simulink model "Newton_Euler_1_D"  (R2023b)
settings: Solver=FixedStepAuto  StartTime=0.0  StopTime=15  RelTol=1e-3  AbsTol=1e-3  EnableMultiTasking=on
model workspace (MAT data in the model file):
  l1 = 20
  m1 = 1
undefined symbols (not defined in the file): X, Y, Z
libraries: sm_lib x13, nesl_utility x13, robotcorelib x1, simulink x1
settings Model: Creator=digimax  LastModifiedBy=digimax
settings SolverCC: AutoScaleAbsTol=off  AlgebraicLoopSolver=TrustRegion  MaxZcPerStep=1
settings DataIOCC: LimitDataPoints=on  MaxDataPoints=10000
settings OptimizationCC: ReuseModelBlockBuffer=off  LifeSpan=inf
settings DebuggingCC: UnconnectedInputMsg=warning  UnconnectedOutputMsg=warning  UnconnectedLineMsg=warning  AllowSymbolicDim=off  SFUnexpectedBacktrackingDiag=warning  SFNoUnconditionalDefaultTransitionDiag=warning  SFExecutionAtInitializationDiag=none  ArithmeticOperatorsInVariantConditions=warning
settings ModelReferenceCC: EnableRefExpFcnMdlSchedulingChecks=on
settings SFSimCC: SimUseLocalCustomCode=off  CustomCodeUndefinedFunction=UseInterfaceOnly
settings RTWCC: RTWUseLocalCustomCode=off  DLArmComputeVersion=19.05
settings CodeAppCC: StateflowObjectComments=on
settings GRTTargetCC: TargetLangStandard=C89/C90 (ANSI)
settings ConfigComp: CovMetricSettings=dw  CovSaveCumulativeToWorkspaceVar=on  CovSaveSingleToWorkspaceVar=on  CovExternalEMLEnable=off  CovSFcnEnable=off
settings SimscapeCC: SimscapeLogType=all  SimscapeLogSimulationStatistics=on  SimscapeLogDataHistory=10000

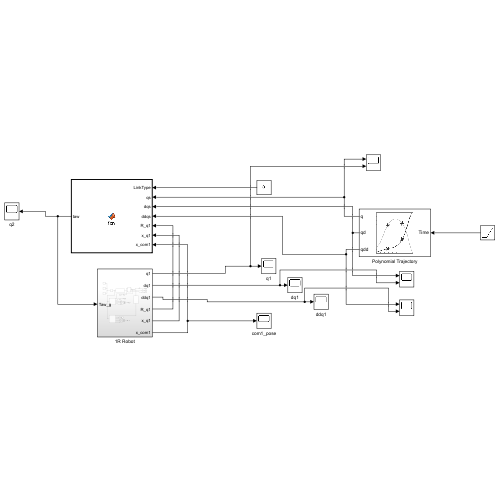
[thumbnail: Simulink's stored preview of the top-level diagram]
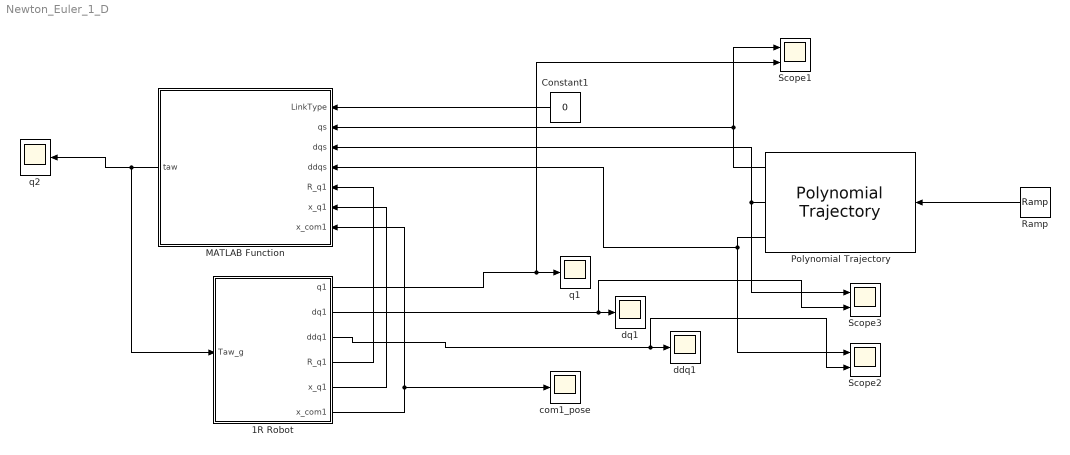
== system Newton_Euler_1_D ==
  1R Robot : Subsystem
  Constant1 : Constant  Value=0
  MATLAB Function : MATLAB Function  TreatAsAtomicUnit=on
  Polynomial Trajectory : robotcorelib/Polynomial Trajectory  WaypointSource=Internal  Waypoints=[ 0, pi/6,-pi/6 ]  TimePoints=[ 0, 5,10]  TimeInterval=[ 1, 4 ]  Method=Cubic Polynomial  ParameterSource=Internal  VelocityBoundaryCondition=zeros( 1, 3)  AccelerationBoundaryCondition=zeros( 2, 5 )  SimulateUsing=Interpreted execution
  Ramp : simulink/Sources/Ramp  slope=1  start=0  InitialOutput=0
  Scope1 : Scope  NumInputPorts=2
  Scope2 : Scope  NumInputPorts=2
  Scope3 : Scope  NumInputPorts=2
  com1_pose : Scope
  ddq1 : Scope
  dq1 : Scope
  q1 : Scope
  q2 : Scope
  wires:
  1R Robot/1(q1) -> Scope1/2, q1/1
  1R Robot/6(x_com1) -> MATLAB Function/7(x_com1), com1_pose/1
  1R Robot/4(R_q1) -> MATLAB Function/5(R_q1)
  1R Robot/5(x_q1) -> MATLAB Function/6(x_q1)
  1R Robot/2(dq1) -> Scope3/2, dq1/1
  Constant1/1 -> MATLAB Function/1(LinkType)
  Ramp/1 -> Polynomial Trajectory/1
  Polynomial Trajectory/1 -> MATLAB Function/2(qs), Scope1/1
  Polynomial Trajectory/2 -> MATLAB Function/3(dqs), Scope3/1
  1R Robot/3(ddq1) -> Scope2/2, ddq1/1
  Polynomial Trajectory/3 -> MATLAB Function/4(ddqs), Scope2/1
  MATLAB Function/1(taw) -> 1R Robot/1(Taw_g), q2/1

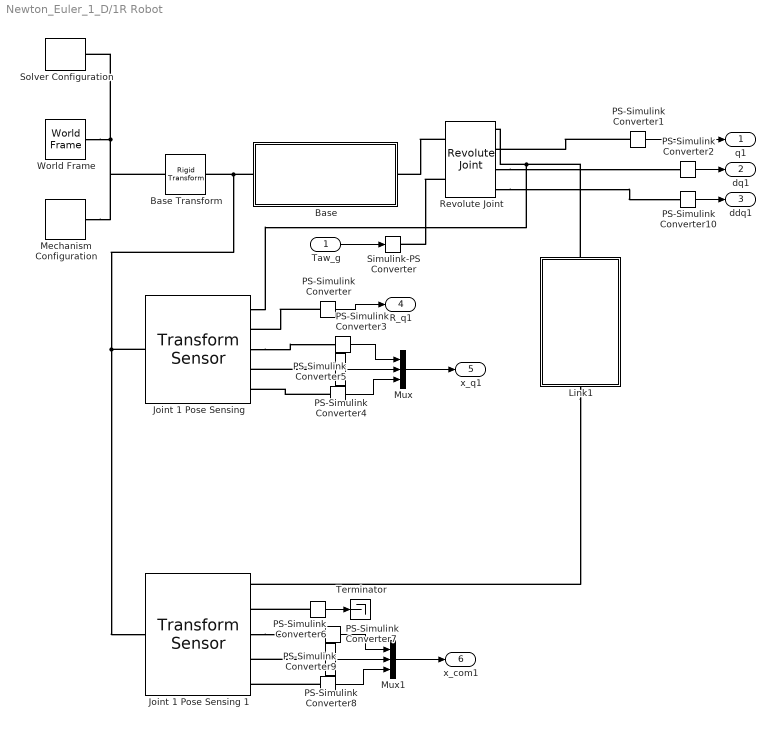
== system Newton_Euler_1_D/1R Robot ==
  Taw_g : Inport
  Base : Subsystem
  Base Transform : sm_lib/Frames and Transforms/Rigid Transform  TranslationMethod=None  TranslationStandardOffset=0  TranslationStandardOffsetUnits=m  TranslationStandardAxis=+Z  TranslationCartesianOffset=[0 0 0]  TranslationCartesianOffsetUnits=m  TranslationROffset=0  TranslationROffsetUnits=m  TranslationZOffset=0  TranslationZOffsetUnits=m  TranslationThetaOffset=0  TranslationThetaOffsetUnits=deg  RotationMethod=AlignedAxes  RotationAngleUnits=deg  RotationStandardAxis=+Z  RotationAngle=0.0  RotationArbitraryAxis=[0 0 1]  FollAlignAxisA=+Z  BaseAlignAxisA=-Y  FollAlignAxisB=+X  BaseAlignAxisB=+X  RotationSequenceAxes=FollowerAxes  RotationSequence=XYX  RotationSequenceAngles=[0 0 0]  RotationSequenceAnglesUnits=deg  RotationMatrix=[1 0 0; 0 1 0; 0 0 1]  Quaternion=[1 0 0 0]
  "Joint 1 Pose Sensing " : sm_lib/Frames and Transforms/Transform Sensor  MeasurementFrame=Base  RotationSequence=XYX  SenseAngle=off  SenseAxis=off  SenseQ=off  SenseR=on  SenseRotationSequence=off  SenseOmegaX=off  SenseOmegaY=off  SenseOmegaZ=off  SenseOmega=off  SenseQDot=off  SenseRDot=off  SenseRotationSequenceDot=off  SenseAlphaX=off  SenseAlphaY=off  SenseAlphaZ=off  SenseAlpha=off  SenseQDDot=off  SenseRDDot=off  SenseX=on  SenseY=on  SenseZ=on  SenseXYZ=off  SenseRad=off  SenseAzim=off  SenseDist=off  SenseInc=off  SenseXDot=off  SenseYDot=off  SenseZDot=off  SenseXYZDot=off  SenseRadDot=off  SenseAzimDot=off  SenseDistDot=off  SenseIncDot=off  SenseXDDot=off  SenseYDDot=off  SenseZDDot=off  SenseXYZDDot=off  SenseRadDDot=off  SenseAzimDDot=off  SenseDistDDot=off  SenseIncDDot=off
  Joint 1 Pose Sensing 1 : sm_lib/Frames and Transforms/Transform Sensor  MeasurementFrame=Base  RotationSequence=XYX  SenseAngle=off  SenseAxis=off  SenseQ=off  SenseR=on  SenseRotationSequence=off  SenseOmegaX=off  SenseOmegaY=off  SenseOmegaZ=off  SenseOmega=off  SenseQDot=off  SenseRDot=off  SenseRotationSequenceDot=off  SenseAlphaX=off  SenseAlphaY=off  SenseAlphaZ=off  SenseAlpha=off  SenseQDDot=off  SenseRDDot=off  SenseX=on  SenseY=on  SenseZ=on  SenseXYZ=off  SenseRad=off  SenseAzim=off  SenseDist=off  SenseInc=off  SenseXDot=off  SenseYDot=off  SenseZDot=off  SenseXYZDot=off  SenseRadDot=off  SenseAzimDot=off  SenseDistDot=off  SenseIncDot=off  SenseXDDot=off  SenseYDDot=off  SenseZDDot=off  SenseXYZDDot=off  SenseRadDDot=off  SenseAzimDDot=off  SenseDistDDot=off  SenseIncDDot=off
  Link1 : Subsystem
  Mechanism Configuration : sm_lib/Utilities/Mechanism Configuration  UniformGravity=Constant  GravityVector=[0 0 -9.81]  GravityVectorUnits=m/s^2  LinearizationDelta=0.001  JointModeTransitionNonlinearIterations=2
  Mux : Mux  Inputs=3
  Mux1 : Mux  Inputs=3
  PS-Simulink Converter{,1..10} (11 alike) : nesl_utility/PS-Simulink Converter  PhysicalDomain=network_engine_domain  SubClassName=ps_output  LeftPortType=input  RightPortType=output  PseudoPeriodic=off  Frequencies=[]  VectorFormat=inherit  Unit=inherit  AffineConversion=off
  Revolute Joint : sm_lib/Joints/Revolute Joint  JointMode=Normal  SenseConstraintForce=off  SenseConstraintForceX=off  SenseConstraintForceY=off  SenseConstraintForceZ=off  SenseConstraintTorque=off  SenseConstraintTorqueX=off  SenseConstraintTorqueY=off  SenseConstraintTorqueZ=off  SenseTotalForce=off  SenseTotalForceX=off  SenseTotalForceY=off  SenseTotalForceZ=off  SenseTotalTorque=off  SenseTotalTorqueX=off  SenseTotalTorqueY=off  SenseTotalTorqueZ=off  CompositeWrenchDir=FollowerOnBase  CompositeWrenchFrame=BaseFrame  EquilibriumPosition=0  EquilibriumPositionUnits=deg  SpringStiffness=0  SpringStiffnessUnits=N*m/deg  DampingCoefficient=0  DampingCoefficientUnits=N*m/(deg/s)  TorqueActuationMode=InputTorque  MotionActuationMode=ComputedMotion  SensePosition=on  SenseVelocity=on  SenseAcceleration=on  SenseTorqueForce=off  SenseLowerLimitTorqueForce=off  SenseUpperLimitTorqueForce=off  LowerLimitSpecify=off  LowerLimitBound=-90  LowerLimitBoundUnits=deg  LowerLimitStiffness=1e4  LowerLimitStiffnessUnits=N*m/deg  LowerLimitDamping=10  LowerLimitDampingUnits=N*m/(deg/s)  LowerLimitTransitionRegionWidth=0.1  LowerLimitTransitionRegionWidthUnits=deg  UpperLimitSpecify=off  UpperLimitBound=90  UpperLimitBoundUnits=deg  UpperLimitStiffness=1e4  UpperLimitStiffnessUnits=N*m/deg  UpperLimitDamping=10  UpperLimitDampingUnits=N*m/(deg/s)  UpperLimitTransitionRegionWidth=0.1  UpperLimitTransitionRegionWidthUnits=deg  PositionTargetSpecify=on  PositionTargetPriority=High  PositionTargetValue=0  PositionTargetValueUnits=deg  VelocityTargetSpecify=off  VelocityTargetPriority=High  VelocityTargetValue=0  VelocityTargetValueUnits=deg/s
  Simulink-PS Converter : nesl_utility/Simulink-PS Converter  PhysicalDomain=network_engine_domain  SubClassName=ps_input  LeftPortType=input  RightPortType=output  PseudoPeriodic=off  Frequencies=[]  NoiseDistribution=none  NoiseParameters=[]  Unit=1  AffineConversion=off  FilteringAndDerivatives=provide  SimscapeFilterOrder=1  InputFilterTimeConstant=0.001  UdotUserProvided=0
  Solver Configuration : nesl_utility/Solver Configuration  PhysicalDomain=network_engine_domain  SubClassName=solver  LeftPortType=input  RightPortType=generic  Tones=[]  Harmonics=[]  SimulateNoise=off  Profile=off  UseLocalSampling=off  EnableSwitchedLinearOptims=on  FrequencyDomain=off  UseCCode=off  RelTol=0.001  AbsTol=1e-06  MinStep=1e-09  ToWorkspace=off  RevertToSquareIcSolve=off  NumHomotopyIterations=100  PhasorMode=off  PhasorModeNumHarmonics=1  ConsistencySolver=NEWTON_XTOL_AFTER_FTOL  IndexReductionMethod=DerivativeReplacement  DoDC=off  ResidualTolerance=1e-09  ConsistencyTolSource=GLOBAL  ConsistencyAbsTol=0.001  ConsistencyRelTol=0.001  ConsistencyTolFactor=0.001  UseLocalSolver=off  LocalSolverChoice=NE_BACKWARD_EULER_ADVANCER  ResolveIndetEquations=on  FunctionEvalNumThread=1  LocalSolverSampleTime=0.001  DoFixedCost=off  MaxNonlinIter=3  MaxModeIter=2  ComputeImpulses=off  ImpulseIterations=2  LinearAlgebra=Sparse  LinearAlgebraNumThread=0  EquationFormulation=NE_TIME_EF  DelaysMemoryBudget=1024  AutomaticFiltering=on  FilteringTimeConstant=0.001  PartitionStorageMethod=AS_NEEDED  PartitionMemoryBudget=1024  PartitionMethod=FAST  MultibodyUseLocalSolver=off  MultibodyLocalSolverChoice=ODE1  MultibodyLocalSolverSampleTime=0.001
  Terminator : Terminator
  World Frame : sm_lib/Frames and Transforms/World Frame
  q1 : Outport
  dq1 : Outport  Port=2
  ddq1 : Outport  Port=3
  R_q1 : Outport  Port=4
  x_q1 : Outport  Port=5
  x_com1 : Outport  Port=6
  wires:
  PS-Simulink Converter1/1 -> q1/1
  Taw_g/1 -> Simulink-PS Converter/1
  PS-Simulink Converter/1 -> R_q1/1
  PS-Simulink Converter3/1 -> Mux/1
  PS-Simulink Converter4/1 -> Mux/2
  PS-Simulink Converter5/1 -> Mux/3
  Mux/1 -> x_q1/1
  Mux1/1 -> x_com1/1
  PS-Simulink Converter9/1 -> Mux1/3
  PS-Simulink Converter8/1 -> Mux1/2
  PS-Simulink Converter7/1 -> Mux1/1
  PS-Simulink Converter6/1 -> Terminator/1
  PS-Simulink Converter10/1 -> ddq1/1
  PS-Simulink Converter2/1 -> dq1/1
  connections:
  Revolute Joint/LConn1 -- Base/RConn1
  PS-Simulink Converter1/LConn1 -- Revolute Joint/RConn2
  Link1/LConn1 -- Revolute Joint/RConn1 -- "Joint 1 Pose Sensing "/RConn1
  Revolute Joint/LConn2 -- Simulink-PS Converter/RConn1
  PS-Simulink Converter/LConn1 -- "Joint 1 Pose Sensing "/RConn2
  "Joint 1 Pose Sensing "/RConn3 -- PS-Simulink Converter3/LConn1
  PS-Simulink Converter4/LConn1 -- "Joint 1 Pose Sensing "/RConn4
  PS-Simulink Converter8/LConn1 -- Joint 1 Pose Sensing 1/RConn4
  PS-Simulink Converter9/LConn1 -- Joint 1 Pose Sensing 1/RConn5
  PS-Simulink Converter6/LConn1 -- Joint 1 Pose Sensing 1/RConn2
  Joint 1 Pose Sensing 1/RConn3 -- PS-Simulink Converter7/LConn1
  Link1/RConn1 -- Joint 1 Pose Sensing 1/RConn1
  PS-Simulink Converter5/LConn1 -- "Joint 1 Pose Sensing "/RConn5
  World Frame/RConn1 -- Base Transform/LConn1 -- Mechanism Configuration/RConn1 -- Solver Configuration/RConn1
  Base/LConn1 -- Joint 1 Pose Sensing 1/LConn1 -- "Joint 1 Pose Sensing "/LConn1 -- Base Transform/RConn1
  Revolute Joint/RConn3 -- PS-Simulink Converter2/LConn1
  Revolute Joint/RConn4 -- PS-Simulink Converter10/LConn1

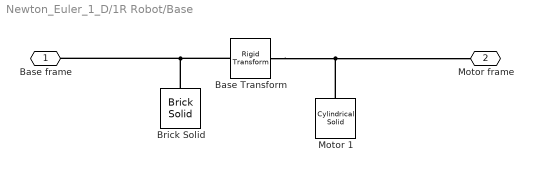
== system Newton_Euler_1_D/1R Robot/Base ==
  Base Transform : sm_lib/Frames and Transforms/Rigid Transform  TranslationMethod=StandardAxis  TranslationStandardOffset=2  TranslationStandardOffsetUnits=m  TranslationStandardAxis=+Z  TranslationCartesianOffset=[0 0 0]  TranslationCartesianOffsetUnits=m  TranslationROffset=0  TranslationROffsetUnits=m  TranslationZOffset=0  TranslationZOffsetUnits=m  TranslationThetaOffset=0  TranslationThetaOffsetUnits=deg  RotationMethod=None  RotationAngleUnits=deg  RotationStandardAxis=+Z  RotationAngle=0.0  RotationArbitraryAxis=[0 0 1]  FollAlignAxisA=+Z  BaseAlignAxisA=-Y  FollAlignAxisB=+X  BaseAlignAxisB=+X  RotationSequenceAxes=FollowerAxes  RotationSequence=XYX  RotationSequenceAngles=[0 0 0]  RotationSequenceAnglesUnits=deg  RotationMatrix=[1 0 0; 0 1 0; 0 0 1]  Quaternion=[1 0 0 0]
  Brick Solid : sm_lib/Body Elements/Brick Solid  GraphicAmbientColor=[0.15 0.15 0.15 1.0]  BasedOnType=Mass  BrickDimensions=[10 10 1]  BrickDimensionsUnits=m  CenterOfMass=[0 0 0]  CenterOfMassUnits=m  GraphicDiffuseColor=[0.5 0.5 0.5]  Density=1000  DensityUnits=kg/m^3  DoExposeReferenceFrame=on  GraphicEmissiveColor=[0.0 0.0 0.0 1.0]  ExportEntireGeometry=off  SerializedFrames=<Frames/>  MarkerShape=Sphere  MarkerSize=10  GraphicType=FromGeometry  InertiaType=CalculateFromGeometry  Mass=1  MassUnits=kg  MomentsOfInertia=[1 1 1]  MomentsOfInertiaUnits=kg*m^2  GraphicOpacity=1.0  ProductsOfInertia=[0 0 0]  ProductsOfInertiaUnits=kg*m^2  GraphicShininess=75  GraphicSpecularColor=[0.5 0.5 0.5 1.0]  GraphicVisPropType=SimpleVisualProperties
  Motor 1 : sm_lib/Body Elements/Cylindrical Solid  GraphicAmbientColor=[0.15 0.15 0.15 1.0]  BasedOnType=Mass  CenterOfMass=[0 0 0]  CenterOfMassUnits=m  GraphicDiffuseColor=[0.4 0.4 0.4]  CylinderLength=3  CylinderLengthUnits=m  CylinderRadius=1  CylinderRadiusUnits=m  Density=1000  DensityUnits=kg/m^3  DoExposeReferenceFrame=on  GraphicEmissiveColor=[0.0 0.0 0.0 1.0]  ExportEntireGeometry=off  SerializedFrames=<Frames/>  MarkerShape=Sphere  MarkerSize=10  GraphicType=FromGeometry  InertiaType=CalculateFromGeometry  Mass=1  MassUnits=kg  MomentsOfInertia=[1 1 1]  MomentsOfInertiaUnits=kg*m^2  GraphicOpacity=1.0  ProductsOfInertia=[0 0 0]  ProductsOfInertiaUnits=kg*m^2  GraphicShininess=75  GraphicSpecularColor=[0.5 0.5 0.5 1.0]  GraphicVisPropType=SimpleVisualProperties
  Base frame : PMIOPort  Side=Left
  Motor frame : PMIOPort  Port=2  Side=Right
  connections:
  Brick Solid/RConn1 -- Base Transform/LConn1 -- Base frame/RConn1
  Base Transform/RConn1 -- Motor 1/RConn1 -- Motor frame/RConn1

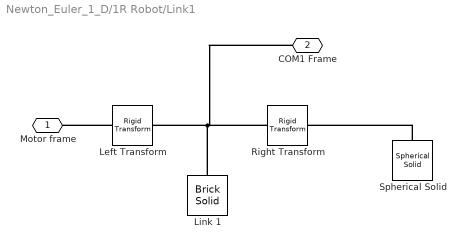
== system Newton_Euler_1_D/1R Robot/Link1 ==
  Left Transform : sm_lib/Frames and Transforms/Rigid Transform  TranslationMethod=StandardAxis  TranslationStandardOffset=10  TranslationStandardOffsetUnits=m  TranslationStandardAxis=+X  TranslationCartesianOffset=[0 0 0]  TranslationCartesianOffsetUnits=m  TranslationROffset=0  TranslationROffsetUnits=m  TranslationZOffset=0  TranslationZOffsetUnits=m  TranslationThetaOffset=0  TranslationThetaOffsetUnits=deg  RotationMethod=None  RotationAngleUnits=deg  RotationStandardAxis=+Z  RotationAngle=0.0  RotationArbitraryAxis=[0 0 1]  FollAlignAxisA=+Z  BaseAlignAxisA=-Y  FollAlignAxisB=+X  BaseAlignAxisB=+X  RotationSequenceAxes=FollowerAxes  RotationSequence=XYX  RotationSequenceAngles=[0 0 0]  RotationSequenceAnglesUnits=deg  RotationMatrix=[1 0 0; 0 1 0; 0 0 1]  Quaternion=[1 0 0 0]
  Link 1 : sm_lib/Body Elements/Brick Solid  GraphicAmbientColor=[0.15 0.15 0.15 1.0]  BasedOnType=Mass  BrickDimensions=[20 1 1]  BrickDimensionsUnits=m  CenterOfMass=[0 0 0]  CenterOfMassUnits=m  GraphicDiffuseColor=[1.0 0.0 0.0]  Density=1000  DensityUnits=kg/m^3  DoExposeReferenceFrame=on  GraphicEmissiveColor=[0.0 0.0 0.0 1.0]  ExportEntireGeometry=off  SerializedFrames=<Frames/>  MarkerShape=Sphere  MarkerSize=10  GraphicType=FromGeometry  InertiaType=CalculateFromGeometry  Mass=1  MassUnits=kg  MomentsOfInertia=[1 1 1]  MomentsOfInertiaUnits=kg*m^2  GraphicOpacity=1.0  ProductsOfInertia=[0 0 0]  ProductsOfInertiaUnits=kg*m^2  GraphicShininess=75  GraphicSpecularColor=[0.5 0.5 0.5 1.0]  GraphicVisPropType=SimpleVisualProperties
  "Right Transform " : sm_lib/Frames and Transforms/Rigid Transform  TranslationMethod=StandardAxis  TranslationStandardOffset=10  TranslationStandardOffsetUnits=m  TranslationStandardAxis=+X  TranslationCartesianOffset=[0 0 0]  TranslationCartesianOffsetUnits=m  TranslationROffset=0  TranslationROffsetUnits=m  TranslationZOffset=0  TranslationZOffsetUnits=m  TranslationThetaOffset=0  TranslationThetaOffsetUnits=deg  RotationMethod=None  RotationAngleUnits=deg  RotationStandardAxis=+Z  RotationAngle=0.0  RotationArbitraryAxis=[0 0 1]  FollAlignAxisA=+Z  BaseAlignAxisA=-Y  FollAlignAxisB=+X  BaseAlignAxisB=+X  RotationSequenceAxes=FollowerAxes  RotationSequence=XYX  RotationSequenceAngles=[0 0 0]  RotationSequenceAnglesUnits=deg  RotationMatrix=[1 0 0; 0 1 0; 0 0 1]  Quaternion=[1 0 0 0]
  Spherical Solid : sm_lib/Body Elements/Spherical Solid  GraphicAmbientColor=[0.15 0.15 0.15 1.0]  BasedOnType=Mass  CenterOfMass=[0 0 0]  CenterOfMassUnits=m  GraphicDiffuseColor=[0.0 0.0 0.8]  Density=1000  DensityUnits=kg/m^3  DoExposeReferenceFrame=on  GraphicEmissiveColor=[0.0 0.0 0.0 1.0]  ExportEntireGeometry=off  SerializedExposedGeometries=<ExposedGeometries/>  SerializedFrames=<Frames/>  MarkerShape=Sphere  MarkerSize=10  GraphicType=FromGeometry  InertiaType=CalculateFromGeometry  Mass=0  MassUnits=kg  MomentsOfInertia=[1 1 1]  MomentsOfInertiaUnits=kg*m^2  GraphicOpacity=1.0  ProductsOfInertia=[0 0 0]  ProductsOfInertiaUnits=kg*m^2  GraphicShininess=75  GraphicSpecularColor=[0.5 0.5 0.5 1.0]  SphereRadius=1  SphereRadiusUnits=m  GraphicVisPropType=SimpleVisualProperties
  Motor frame : PMIOPort  Side=Left
  COM1 Frame : PMIOPort  Port=2  Side=Right
  connections:
  Link 1/RConn1 -- "Right Transform "/LConn1 -- COM1 Frame/RConn1 -- Left Transform/RConn1
  Left Transform/LConn1 -- Motor frame/RConn1
  Spherical Solid/RConn1 -- "Right Transform "/RConn1

== matlab function Newton_Euler_1_D/MATLAB Function ==
  data: LinkType input; qs input; dqs input; ddqs input; R_q1 input; x_q1 input; x_com1 input; taw output
function taw = fcn(LinkType , qs , dqs, ddqs , R_q1 , x_q1 , x_com1)

    % Characteristics 
    linkType = [0;LinkType] ; 

    Link_num = length(LinkType) ;   % Number of Links
 
    m = zeros(Link_num+1 , 1) ;    % Vector of link masses
    m(2) = 1 ; % unit kg

    g = 9.81 ; 

    % dimensions of the links in its body frame 
    x= 20;
    y = 1 ; 
    z = 1 ; 


    Ix = m(2)/12*(x^2) ; 
    Iy = m(2)/12*(x^2) ;
    Iz = m(2)/12*(x^2) ;

    Ic1_1 = [Ix 0 0;
            0 Iy 0;
            0 0 Iz] ; 

    Ic_i = zeros(3,3,Link_num+1) ;  % matrix of inertias in the frame connected to its joint
    Ic_i(:,:,2) = Ic1_1 ; 

    
    %% Initialization 

    ri_0_0 = [zeros(3,1),x_q1];                             % Position of Joint i w.r.t base frame represented in base frame  
    r_ci_0_0 = [zeros(3,1),x_com1] ;                        % Position of Link i C.M w.r.t base frame represented in base frame  
    r_i_i_1_0 = zeros(3,Link_num+1) ;                       % Position of Joint i w.r.t Joint i-1 represented in base frame
    P_ci_i_0 = zeros(3,Link_num+1) ;

    % Matrices of Rotation
    R0_i =  zeros(3,3,Link_num+1);                      
    R0_i(:,:,1) = eye(3) ;
    R0_i(:,:,2) = R_q1 ;
    
    
    
    wi_0_i = zeros(3,Link_num+1) ;      % Vector of angular velocities of join i w.r.t base frame presented in frame i 
    vi_0_0 = zeros(3,Link_num+1) ;      % Vector of Linear velocities of link i w.r.t base frame presented in frame i
    vci_0_0 = zeros(3,Link_num+1) ;     % Vector of Linear velocities of link i COM w.r.t base frame presented in frame i

    q = [0 , qs.'];                       % Vector of Joint movement
    dq = [0 , dqs.'];                     % Vector of Joint velocity
    ddq = [0 , ddqs.'];                   % Vector of Joint acceleration

    dwi_0_i = zeros(3,Link_num+1) ;     % Vector of angular acceleration of join i w.r.t base frame presented in base frame 
    dvi_0_i = zeros(3,Link_num+1) ;     % Vector of Linear acceleration of link i w.r.t base frame presented in base frame
    dvi_0_i(:,1) = [0;g;0] ;
    dvci_0_i = zeros(3,Link_num+1) ;    % Vector of Linear acceleration of link i COM w.r.t base frame presented in base frame


    Fci_i = zeros(3, Link_num+1) ;      % Vector of Forces applied to Link i COM presented in base frame 
    Nci_i = zeros(3, Link_num+1) ;      % Vector of Torques applied to Link i COM presented in base frame   

    % Initialize forces and torques on the end-effector
    fee=[0;0;0];
    nee=[0;0;0];


    taw = [0] ; 

    %% Forward recursive 


    %% Velocity 

    for i = 2 : Link_num+1

        if linkType(i) == 0

            r_i_i_1_0(:,i) = ri_0_0(:,i) - ri_0_0(:,i-1) ;  % position vector of joint i w.r.t joint i-1 represented in base frame

            wi_0_i(:,i) = R0_i(:,:,i).'*R0_i(:,:,i-1)*wi_0_i(:,i-1) + R0_i(:,:,i).'*R0_i(:,3,i)*dq(i) ; 
        
        elseif linkType(i) == 1

            r_i_i_1_0(:,i) = ri_0_0(:,i) - ri_0_0(:,i-1) ;  % position vector of joint i w.r.t joint i-1 represented in base frame

            wi_0_i(:,i) = R0_i(:,:,i).'*R0_i(:,:,i-1)*wi_0_i(:,i-1);


        end
         
    end



    %% Acceleration 

    for i = 2:Link_num+1

        if linkType(i) ==0

            dwi_0_i(:,i) = R0_i(:,:,i).'*R0_i(:,:,i-1)*dwi_0_i(:,i-1) + cross(R0_i(:,:,i).'*R0_i(:,:,i-1)*wi_0_i(:,i-1) , R0_i(:,:,i).'*R0_i(:,3,i)*dq(i)) ...
                + R0_i(:,:,i).'*R0_i(:,3,i)*ddq(i) ; 
            dvi_0_i(:,i) = R0_i(:,:,i).'*R0_i(:,:,i-1)*(dvi_0_i(:,i-1) + cross(dwi_0_i(:,i-1) , R0_i(:,:,i-1).'*r_i_i_1_0(:,i)) ...
                + cross(wi_0_i(:,i-1) , cross(wi_0_i(:,i-1) , R0_i(:,:,i-1).'*r_i_i_1_0(:,i)))) ;  


        elseif linkType(i) == 1

            dwi_0_i(:,i) = R0_i(:,:,i).'*R0_i(:,:,i-1)*dwi_0_i(:,i-1) ;
            dvi_0_i(:,i) = R0_i(:,:,i).'*R0_i(:,:,i-1)*(dvi_0_i(:,i-1) + cross(dwi_0_i(:,i-1) , R0_i(:,:,i-1).'*r_i_i_1_0(:,i)) ...
                + cross(wi_0_i(:,i-1) , cross(wi_0_i(:,i-1) , R0_i(:,:,i-1).'*r_i_i_1_0(:,i))))...
                + 2*cross(R0_i(:,:,i).'*R0_i(:,:,i-1)*wi_0_i(:,i-1) , R0_i(:,:,i).'*R0_i(:,3,i)*dq(i)) + R0_i(:,:,i).'*R0_i(:,3,i)*ddq(i);  

        end

        P_ci_i_0 (:,i) = r_ci_0_0(:,i)-ri_0_0(:,i) ;  % Location of lonk i C.M wrt to its joint location presented in abse frame 
        dvci_0_i(:,i) = dvi_0_i(:,i) + cross(dwi_0_i(:,i) , R0_i(:,:,i).'*P_ci_i_0 (:,i)) + cross(wi_0_i(:,i) , cross(wi_0_i(:,i) , R0_i(:,:,i).'*P_ci_i_0 (:,i))) ;  


    end
    
   
    %% Force on C.M


    for i = 2:Link_num+1

        Fci_i(:,i) = m(i)*dvci_0_i(:,i) ;
        Nci_i(:,i) = Ic_i(:,:,i) * dwi_0_i(:,i) + cross(wi_0_i(:,i), Ic_i(:,:,i) *wi_0_i(:,i)) ; 


    end


    %% Backward Recursion 

    F_i = zeros(3,Link_num + 1) ;
    N_i = zeros(3,Link_num + 1) ;
    
    % Link 1
    % Rotational
    F_i(:,2) = Fci_i(:,2) ; 

    N_i(:,2) = Nci_i(:,2) +  cross(R0_i(:,:,2).'*P_ci_i_0 (:,2) , Fci_i(:,2)) ;    

    
    

    taw = N_i(:,2).' *R0_i(:,:,2).'*R0_i(:,3,2) ;
      
    
    
end
